simulink library "platooning_custom_blocks"  (R2018b)
settings: Solver=VariableStepAuto  StartTime=0.0  StopTime=10.0  RelTol=1e-3
undefined symbols (not defined in the file): AccPdl_pdlbpt, AccPdl_spdbpt, AccPdl_trqMap, adj_motEffMap, BETModel, BrkPdl_brkTrq, BrkPdl_pdlbpt, Cd_Map, Cd_Map_T2, CT_accPdl_pdlbpt, CT_accPdl_spdbpt, CT_accPdl_trqMap, CT_brkPdl_brkTrq, CT_brkPdl_pdlbpt, CTModel, d_11, d_22, DiscIntNeverNeededParam, init_veh_spd_mps, max_Cd_frac, min_Cd_frac, motSpdVec, motTrqVec, msk_init_pos_m, msk_mot_cont_trq, msk_mot_num, msk_mot_spd_bpt, N_OptResults, sim_t_step, simDrv, SPHETModel, t_step
libraries: simulink x19, $bdroot x16, dspstat3 x2, custom_func x1
(part 3 of 5)

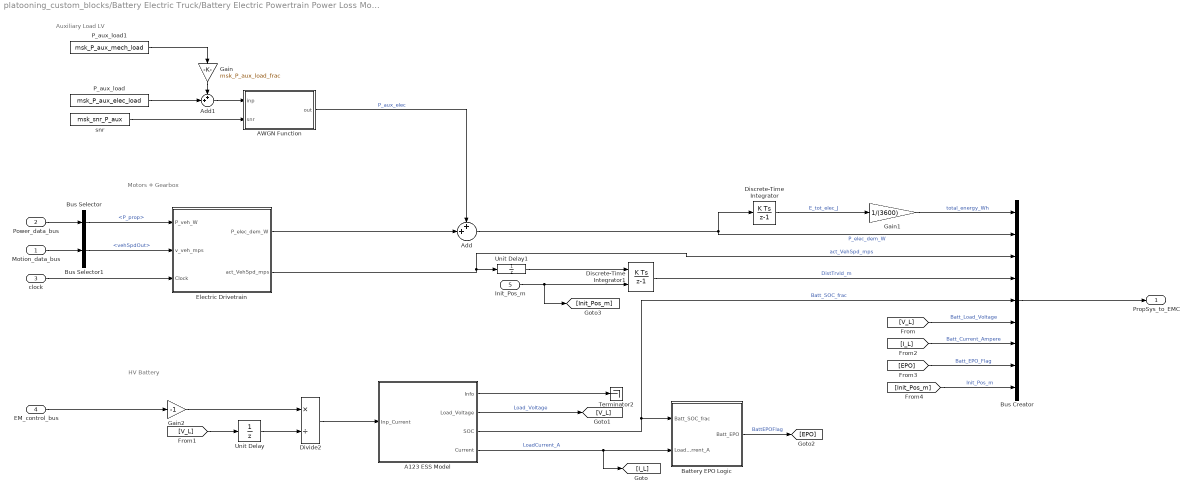
== system platooning_custom_blocks/Battery Electric Truck/Battery Electric Powertrain Power Loss Model ==
  note: Motors + Gearbox
  note: Auxiliary Load LV
  note: HV Battery
  Motion_data_bus : Inport
  Power_data_bus : Inport  Port=2
  clock : Inport  Port=3
  EM_control_bus : Inport  Port=4
  Init_Pos_m : Inport  Port=5
  A123 ESS Model : Subsystem
  AWGN Function : MATLAB Function  TreatAsAtomicUnit=on
  Add : Sum  Inputs=++|
  Add1 : Sum  Inputs=++|
  Battery EPO Logic : Subsystem
  Bus Creator : BusCreator  Inputs=9
  Bus Selector : BusSelector  OutputSignals=P_prop
  Bus Selector1 : BusSelector  OutputSignals=vehSpdOut
  Discrete-Time Integrator : DiscreteIntegrator  SampleTime=msk_t_step  ICPrevOutput=DiscIntNeverNeededParam  ICPrevScaledInput=DiscIntNeverNeededParam
  Discrete-Time Integrator1 : DiscreteIntegrator  InitialConditionSource=external  SampleTime=msk_t_step  ICPrevOutput=DiscIntNeverNeededParam  ICPrevScaledInput=DiscIntNeverNeededParam
  Divide2 : Product  Inputs=*/
  Electric Drivetrain : Subsystem
  Gain : Gain  Gain=msk_P_aux_load_frac
  Gain1 : Gain  Gain=1/(3600)
  Gain2 : Gain  Gain=-1
  P_aux_load : Constant  Value=msk_P_aux_elec_load
  P_aux_load1 : Constant  Value=msk_P_aux_mech_load
  Terminator2 : Terminator
  Unit Delay : UnitDelay  InitialCondition=msk_batt_Ns* msk_batt_Nmod * msk_cell_Vnom  SampleTime=-1
  Unit Delay1 : UnitDelay  SampleTime=-1
  snr : Constant  Value=msk_snr_P_aux
  PropSys_to_EMC : Outport
  wires:
  [Init_Pos_m] -> Bus Creator/9  "Init_Pos_m"
  [EPO] -> Bus Creator/8  "Batt_EPO_Flag"
  [I_L] -> Bus Creator/7  "Batt_Current_Ampere"
  P_aux_load1/1 -> Gain/1
  Gain/1 -> Add1/1
  Add1/1 -> AWGN Function/1(inp)
  Init_Pos_m/1 -> Discrete-Time Integrator1/2, [Init_Pos_m]
  Power_data_bus/1 -> Bus Selector/1
  Motion_data_bus/1 -> Bus Selector1/1
  clock/1 -> Electric Drivetrain/3(Clock)
  Bus Selector1/1 -> Electric Drivetrain/2(v_veh_mps)  "<vehSpdOut>"
  Bus Selector/1 -> Electric Drivetrain/1(P_veh_W)  "<P_prop>"
  P_aux_load/1 -> Add1/2
  snr/1 -> AWGN Function/2(snr)
  AWGN Function/1(out) -> Add/1  "P_aux_elec"
  Add/1 -> Bus Creator/2, Discrete-Time Integrator/1  "P_elec_dem_W"
  Electric Drivetrain/1(P_elec_dem_W) -> Add/2
  Bus Creator/1 -> PropSys_to_EMC/1
  Discrete-Time Integrator/1 -> Gain1/1  "E_tot_elec_J"
  Gain1/1 -> Bus Creator/1  "total_energy_Wh"
  A123 ESS Model/2(Load_Voltage) -> [V_L]  "Load_Voltage"
  Divide2/1 -> A123 ESS Model/1(Inp_Current)
  A123 ESS Model/3(SOC) -> Bus Creator/5, Battery EPO Logic/1(Batt_SOC_frac)  "Batt_SOC_frac"
  A123 ESS Model/1(Info) -> Terminator2/1
  [V_L] -> Unit Delay/1
  Unit Delay/1 -> Divide2/2
  Battery EPO Logic/1(Batt_EPO) -> [EPO]  "BattEPOFlag"
  Gain2/1 -> Divide2/1
  EM_control_bus/1 -> Gain2/1
  A123 ESS Model/4(Current) -> Battery EPO Logic/2(LoadCurrent_A), [I_L]  "LoadCurrent_A"
  Electric Drivetrain/2(act_VehSpd_mps) -> Unit Delay1/1, Bus Creator/3  "act_VehSpd_mps"
  Discrete-Time Integrator1/1 -> Bus Creator/4  "DistTrvld_m"
  Unit Delay1/1 -> Discrete-Time Integrator1/1
  [V_L] -> Bus Creator/6  "Batt_Load_Voltage"

== system platooning_custom_blocks/Battery Electric Truck/Battery Electric Truck Energy Management System ==
  PropSys_to_EMC : Inport
  From_PCL_BUS : Inport  Port=2
  Battery Electric Truck Regen Control Algorithm : MATLAB Function  TreatAsAtomicUnit=on
  Battery Temp degC : Constant  Value=25
  Bus Selector : BusSelector  OutputSignals=P_elec_dem_W,Batt_Load_Voltage,Batt_SOC_frac
  Charge Current Continuous : Lookup_n-D  BreakpointsForDimension1=msk_cell_temp_bpt  BreakpointsForDimension2=msk_soc_bpt  Table=msk_cont_chg_map  InternalRulePriority=Speed  RndMeth=Simplest  InputSameDT=on
  Gain : Gain  Gain=-1
  Multiply : Product
  Terminator : Terminator
  Terminator2 : Terminator
  Unit Delay : UnitDelay  SampleTime=-1
  EMC_to_PropSys : Outport
  wires:
  Bus Selector/2 -> Multiply/1  "<Batt_Load_Voltage>"
  Battery Electric Truck Regen Control Algorithm/1(P_mechbrk_W) -> Terminator2/1
  Charge Current Continuous/1 -> Gain/1
  Battery Electric Truck Regen Control Algorithm/2(P_regenbrk_W) -> EMC_to_PropSys/1  "P_batt_W"
  Bus Selector/1 -> Battery Electric Truck Regen Control Algorithm/1(P_elec_dem)  "<P_elec_dem_W>"
  Bus Selector/3 -> Unit Delay/1  "<Batt_SOC_frac>"
  PropSys_to_EMC/1 -> Bus Selector/1
  From_PCL_BUS/1 -> Terminator/1
  Unit Delay/1 -> Charge Current Continuous/2, Battery Electric Truck Regen Control Algorithm/3(Batt_SOC)
  Multiply/1 -> Battery Electric Truck Regen Control Algorithm/2(P_regen_avail)
  Battery Temp degC/1 -> Charge Current Continuous/1
  Gain/1 -> Multiply/2

== system platooning_custom_blocks/Conventional Truck/Conventional Post-Processing ==
  PropSys_to_EMC : Inport
  Blending Function 1 : Subsystem
  Blending Function 2 : Subsystem
  Bus Creator : BusCreator  Inputs=3
  Bus Creator1 : BusCreator  Inputs=5
  Bus Creator2 : BusCreator  Inputs=3
  Bus Creator3 : BusCreator  Inputs=3
  Bus Selector : BusSelector  OutputSignals=fuelUsed_L,DistTrvld_m,InitPos_m,act_VehSpd_mps,gear_cmd
  Constant1 : Constant  Value=eps
  Distance to Empty Calculator : Subsystem
  Divide1 : Product  Inputs=*/
  Fuel Consumption Calculator : Subsystem
  Fuel LHV energy per volume : Constant  Value=msk_fuel_rho_kgpl * msk_fuel_lhv_kwhpkg
  Product : Product
  Short Term Averaging Function : MATLAB Function  TreatAsAtomicUnit=on
  Short term average distance window - meters : Constant  Value=msk_distwin
  Subtract : Sum  Inputs=+-
  Switch : Switch  Criteria=u2 > Threshold
  kWh2Wh : Gain  Gain=1000
  To_PCL_BUS : Outport
  wires:
  Bus Selector/2 -> Subtract/1, Bus Creator1/2  "<DistTrvld_m>"
  Bus Selector/3 -> Subtract/2  "<InitPos_m>"
  Distance to Empty Calculator/1(estDTE_km) -> Bus Creator1/5  "estDTE_km"
  Constant1/1 -> Switch/3
  Switch/1 -> Divide1/2
  Bus Selector/5 -> Bus Creator1/4  "<gear_cmd>"
  Bus Creator1/1 -> Bus Creator3/3  "State_BUS"
  Subtract/1 -> Fuel Consumption Calculator/2(<DistTrvld_m>), Short Term Averaging Function/3(Dist_Traveled), Switch/2, Switch/1  "DistTrvld_m"
  Divide1/1 -> Blending Function 1/1(runAvgFuelEC_Wh_m), Bus Creator/1  "runAvgElecEC_Wh_m"
  Product/1 -> kWh2Wh/1  "usedFuelEnergy_kWh"
  Short Term Averaging Function/1(STAvg_Wh_m) -> Bus Creator/3, Blending Function 1/3(stAvgFuelEC_Wh_m)  "stAvgElecEC_Wh_m"
  Blending Function 1/1(blndElecEC_Wh_m) -> Bus Creator/2  "blndElecEC_Wh_m"
  Bus Creator/1 -> Bus Creator3/1  "EC_BUS"
  Bus Selector/4 -> Bus Creator1/3  "<act_VehSpd_mps>"
  Fuel LHV energy per volume/1 -> Short Term Averaging Function/2(Fuel_LHV_kWhpL), Product/1
  Short term average distance window - meters/1 -> Short Term Averaging Function/4(Dist_Window)
  PropSys_to_EMC/1 -> Bus Selector/1
  Bus Selector/1 -> Product/2, Fuel Consumption Calculator/1(<fuelUsed_L>), Bus Creator1/1, Distance to Empty Calculator/2(<fuelUsed_L>), Blending Function 2/2(Fuel_Used_L), Blending Function 1/2(Fuel_Used_L), Short Term Averaging Function/1(Fuel_Used_L)  "<fuelUsed_L>"
  kWh2Wh/1 -> Divide1/1
  Short Term Averaging Function/2(STAvg_L_100km) -> Bus Creator2/3, Blending Function 2/3(stAvgFC_L_100km)  "stAvgFC_L_100km"
  Fuel Consumption Calculator/1(FC_Lp100km) -> Bus Creator2/1, Blending Function 2/1(runAvgFC_L_100km)  "runAvgFC_L_100km"
  Blending Function 2/1(blndFC_L_100km) -> Bus Creator2/2, Distance to Empty Calculator/1(blndFC_L_100km)  "blndFC_L_100km"
  Bus Creator2/1 -> Bus Creator3/2  "FC_BUS"
  Bus Creator3/1 -> To_PCL_BUS/1

== system platooning_custom_blocks/Conventional Truck/Conventional Powertrain Energy Management System ==
  PropSys_to_EMC : Inport
  From_PCL_BUS : Inport  Port=2
  Bus Selector : BusSelector  OutputSignals=total_power_W,act_VehSpd_mps
  Optimal Gear Shift Algorithm : $bdroot/Optimal Gear Shift Algorithm  msk_tire_radius_m=CTModel.ld_tire_rad_m  msk_trns_eff_avg=mean(CTModel.gear_eff)  msk_init_gear=1
  Rate Transition : RateTransition  OutPortSampleTime=sim_t_step
  Rate Transition1 : RateTransition  OutPortSampleTime=sim_t_step
  Terminator : Terminator
  EMC_to_PropSys : Outport
  wires:
  Rate Transition1/1 -> Optimal Gear Shift Algorithm/2
  Rate Transition/1 -> Optimal Gear Shift Algorithm/1
  From_PCL_BUS/1 -> Terminator/1
  PropSys_to_EMC/1 -> Bus Selector/1
  Bus Selector/1 -> Rate Transition/1  "<total_power_W>"
  Bus Selector/2 -> Rate Transition1/1  "<act_VehSpd_mps>"
  Optimal Gear Shift Algorithm/1 -> EMC_to_PropSys/1  "opt_gear"

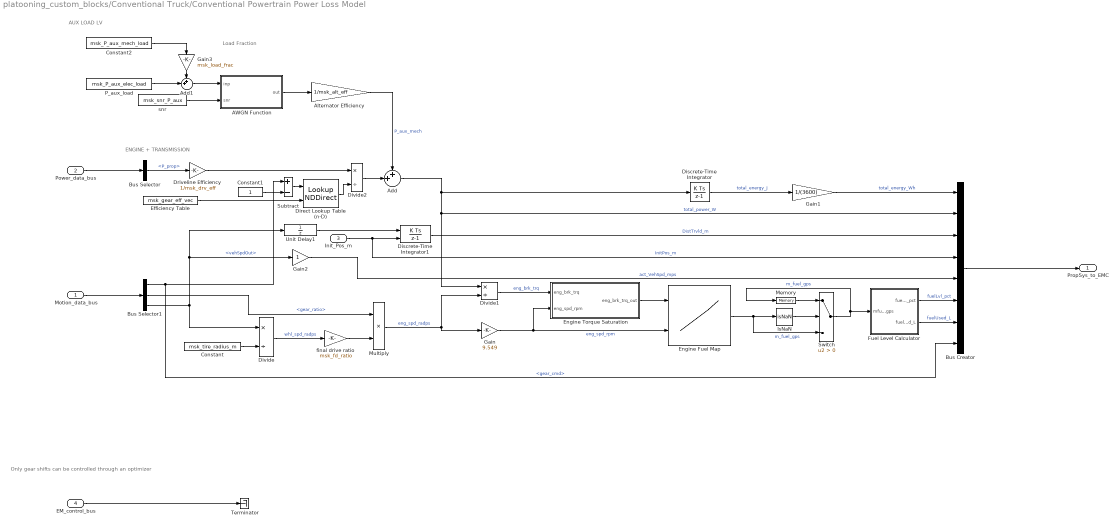
== system platooning_custom_blocks/Conventional Truck/Conventional Powertrain Power Loss Model ==
  note: Only gear shifts can be controlled through an optimizer
  note: ENGINE + TRANSMISSION
  note: AUX LOAD LV
  note: Load Fraction
  Motion_data_bus : Inport
  Power_data_bus : Inport  Port=2
  Init_Pos_m : Inport  Port=3
  EM_control_bus : Inport  Port=4
  AWGN Function : MATLAB Function  TreatAsAtomicUnit=on
  Add : Sum  Inputs=++|
  Add1 : Sum  Inputs=++|
  Alternator Efficiency : Gain  Gain=1/msk_alt_eff
  Bus Creator : BusCreator  Inputs=8
  Bus Selector : BusSelector  OutputSignals=P_prop
  Bus Selector1 : BusSelector  OutputSignals=gear_cmd,gear_ratio,vehSpdOut
  Constant : Constant  Value=msk_tire_radius_m
  Constant1 : Constant
  Constant2 : Constant  Value=msk_P_aux_mech_load
  Direct Lookup Table (n-D) : LookupNDDirect  NumberOfTableDimensions=1  TableIsInput=on
  Discrete-Time Integrator : DiscreteIntegrator  SampleTime=-1  ICPrevOutput=DiscIntNeverNeededParam  ICPrevScaledInput=DiscIntNeverNeededParam
  Discrete-Time Integrator1 : DiscreteIntegrator  InitialConditionSource=external  InitialCondition=msk_init_pos_m  SampleTime=msk_t_step  ICPrevOutput=DiscIntNeverNeededParam  ICPrevScaledInput=DiscIntNeverNeededParam
  Divide : Product  Inputs=*/
  Divide1 : Product  Inputs=*/
  Divide2 : Product  Inputs=*/
  Driveline Efficiency : Gain  Gain=1/msk_drv_eff
  Efficiency Table : Constant  Value=msk_gear_eff_vec
  Engine Fuel Map : Lookup_n-D  BreakpointsForDimension1=msk_eng_trq_bpt  BreakpointsForDimension2=msk_eng_spd_bpt  Table=msk_eng_fuel_map  ExtrapMethod=Clip  UseLastTableValue=on  InternalRulePriority=Speed  RndMeth=Simplest  InputSameDT=on
  Engine Torque Saturation : Subsystem
  Fuel Level Calculator : Subsystem
  Gain : Gain  Gain=9.549
  Gain1 : Gain  Gain=1/(3600)
  Gain2 : Gain
  Gain3 : Gain  Gain=msk_load_frac
  IsNaN : RelationalOperator  Operator=isNaN  OutDataTypeStr=boolean  RndMeth=Simplest
  Memory : Memory
  Multiply : Product
  P_aux_load : Constant  Value=msk_P_aux_elec_load
  Subtract : Sum  Inputs=+-
  Switch : Switch  Criteria=u2 > Threshold
  Terminator : Terminator
  Unit Delay1 : UnitDelay  SampleTime=-1
  final drive ratio : Gain  Gain=msk_fd_ratio
  snr : Constant  Value=msk_snr_P_aux
  PropSys_to_EMC : Outport
  wires:
  P_aux_load/1 -> Add1/2
  Gain3/1 -> Add1/1
  Constant2/1 -> Gain3/1
  Memory/1 -> Switch/1
  IsNaN/1 -> Switch/2
  Engine Fuel Map/1 -> IsNaN/1, Switch/3  "m_fuel_gps"
  Power_data_bus/1 -> Bus Selector/1
  Motion_data_bus/1 -> Bus Selector1/1
  Init_Pos_m/1 -> Discrete-Time Integrator1/2, Bus Creator/4  "InitPos_m"
  EM_control_bus/1 -> Terminator/1
  Bus Selector1/3 -> Gain2/1, Unit Delay1/1, Divide/1  "<vehSpdOut>"
  Bus Selector/1 -> Driveline Efficiency/1  "<P_prop>"
  Add1/1 -> AWGN Function/1(inp)
  snr/1 -> AWGN Function/2(snr)
  AWGN Function/1(out) -> Alternator Efficiency/1
  Alternator Efficiency/1 -> Add/1  "P_aux_mech"
  Switch/1 -> Fuel Level Calculator/1(mfuel_gps), Memory/1  "m_fuel_gps"
  Constant/1 -> Divide/2
  Divide/1 -> final drive ratio/1  "whl_spd_radps"
  final drive ratio/1 -> Multiply/2
  Multiply/1 -> Divide1/2, Gain/1  "eng_spd_radps"
  Gain/1 -> Engine Torque Saturation/2(eng_spd_rpm), Engine Fuel Map/2  "eng_spd_rpm"
  Add/1 -> Bus Creator/2, Divide1/1, Discrete-Time Integrator/1  "total_power_W"
  Divide2/1 -> Add/2
  Bus Selector1/2 -> Multiply/1  "<gear_ratio>"
  Bus Creator/1 -> PropSys_to_EMC/1
  Discrete-Time Integrator/1 -> Gain1/1  "total_energy_J"
  Fuel Level Calculator/1(fuelLvl_pct) -> Bus Creator/6  "fuelLvl_pct"
  Fuel Level Calculator/2(fuelUsed_L) -> Bus Creator/7  "fuelUsed_L"
  Gain1/1 -> Bus Creator/1  "total_energy_Wh"
  Divide1/1 -> Engine Torque Saturation/1(eng_brk_trq)  "eng_brk_trq"
  Engine Torque Saturation/1(eng_brk_trq_out) -> Engine Fuel Map/1
  Unit Delay1/1 -> Discrete-Time Integrator1/1
  Discrete-Time Integrator1/1 -> Bus Creator/3  "DistTrvld_m"
  Gain2/1 -> Bus Creator/5  "act_VehSpd_mps"
  Driveline Efficiency/1 -> Divide2/1
  Efficiency Table/1 -> Direct Lookup Table (n-D)/2
  Direct Lookup Table (n-D)/1 -> Divide2/2
  Subtract/1 -> Direct Lookup Table (n-D)/1
  Constant1/1 -> Subtract/2
  Bus Selector1/1 -> Bus Creator/8, Subtract/1  "<gear_cmd>"

== system platooning_custom_blocks/Series Parallel Hybrid Electric Truck/Series Parallel Hybrid Electric Post-Processing ==
  PropSys_to_EMC : Inport
  Add : Sum
  Battery Energy Max : Constant  Value=msk_batt_Ns * msk_batt_Np * msk_batt_Nmod * msk_cell_Vnom * msk_cell_Q_Ah
  Blending Function 1 : Subsystem
  Blending Function 2 : Subsystem
  Bus Creator1 : BusCreator  Inputs=11
  Bus Creator2 : BusCreator  Inputs=3
  Bus Creator3 : BusCreator  Inputs=3
  Bus Creator5 : BusCreator  Inputs=3
  Bus Selector : BusSelector  OutputSignals=Batt_Voltage_V,Batt_EPO_Flag,Batt_Current_A,P_gen_mech_W,GearCmd,eng_spd_rpm,Batt_SOC_frac,DistTrvld_m,Init_Pos_m,act_VehSpd_mps,fuelUsed_L
  Constant : Constant  Value=msk_batt_soc_init
  Constant2 : Constant  Value=eps
  Distance to Empty Calculator : Subsystem
  Divide1 : Product  Inputs=*/
  Fuel Consumption Calculator : Subsystem
  Fuel LHV energy per volume : Constant  Value=msk_fuel_rho_kgpl * msk_fuel_lhv_kwhpkg
  Product : Product
  Product1 : Product
  Short Term Averaging Function1 : MATLAB Function  TreatAsAtomicUnit=on
  Short term average distance window - meters1 : Constant  Value=msk_distwin
  Subtract : Sum  Inputs=+-
  Subtract1 : Sum  Inputs=+-
  Switch : Switch  Criteria=u2 > Threshold
  kWh2Wh : Gain  Gain=1000
  To_PCL_BUS : Outport
  wires:
  Bus Selector/8 -> Subtract1/1, Bus Creator1/8  "<DistTrvld_m>"
  Bus Selector/9 -> Subtract1/2  "<Init_Pos_m>"
  Bus Selector/6 -> Bus Creator1/6  "<eng_spd_rpm>"
  Bus Selector/5 -> Bus Creator1/5  "<GearCmd>"
  Bus Selector/4 -> Bus Creator1/4  "<P_gen_mech_W>"
  Bus Selector/3 -> Bus Creator1/3  "<Batt_Current_A>"
  Bus Selector/2 -> Bus Creator1/2  "<Batt_EPO_Flag>"
  Bus Selector/1 -> Bus Creator1/1  "<Batt_Voltage_V>"
  Distance to Empty Calculator/1(estDTE_km) -> Bus Creator1/11  "estDTE_km"
  Constant2/1 -> Switch/3
  Switch/1 -> Divide1/2
  PropSys_to_EMC/1 -> Bus Selector/1
  Bus Selector/7 -> Bus Creator1/7, Distance to Empty Calculator/3(battSOC_frac), Short Term Averaging Function1/1(Batt_SOC_frac), Subtract/2  "<Batt_SOC_frac>"
  Constant/1 -> Subtract/1
  Subtract/1 -> Product/2
  Product/1 -> Add/1  "total_elec_Energy_Wh"
  Battery Energy Max/1 -> Short Term Averaging Function1/2(Batt_Max_Energy), Product/1
  Bus Creator1/1 -> Bus Creator2/1  "State_BUS"
  Bus Creator2/1 -> To_PCL_BUS/1
  Bus Creator5/1 -> Bus Creator2/3  "FC_BUS"
  Product1/1 -> kWh2Wh/1  "usedFuelEnergy_kWh"
  Blending Function 2/1(blndFC_L_100km) -> Bus Creator5/2  "blndFC_L_100km"
  Divide1/1 -> Blending Function 1/1(runAvgFuelEC_Wh_m), Bus Creator3/1  "runAvgElecEC_Wh_m"
  Bus Selector/10 -> Bus Creator1/9  "<act_VehSpd_mps>"
  Short Term Averaging Function1/1(STAvg_Wh_m) -> Blending Function 1/3(stAvgFuelEC_Wh_m), Bus Creator3/3  "stAvgElecEC_Wh_m"
  Bus Creator3/1 -> Bus Creator2/2  "EC_BUS"
  Short term average distance window - meters1/1 -> Short Term Averaging Function1/6(Dist_Window)
  Blending Function 1/1(blndElecEC_Wh_m) -> Bus Creator3/2, Distance to Empty Calculator/1(blndEC_Wh_m)  "blndElecEC_Wh_m"
  kWh2Wh/1 -> Add/2
  Subtract1/1 -> Switch/2, Switch/1, Fuel Consumption Calculator/2(<DistTrvld_m>), Short Term Averaging Function1/5(Dist_Traveled)  "DistTrvld_m"
  Short Term Averaging Function1/2(STAvg_L_100km) -> Bus Creator5/3, Blending Function 2/3(stAvgFC_L_100km)  "stAvgFC_L_100km"
  Fuel LHV energy per volume/1 -> Short Term Averaging Function1/4(Fuel_LHV_kWhpL), Product1/1
  Fuel Consumption Calculator/1(FC_Lp100km) -> Bus Creator5/1, Blending Function 2/1(runAvgFC_L_100km)  "runAvgFC_L_100km"
  Bus Selector/11 -> Product1/2, Distance to Empty Calculator/2(<fuelUsed_L>), Blending Function 1/2(Fuel_Used_L), Blending Function 2/2(Fuel_Used_L), Short Term Averaging Function1/3(Fuel_Used_L), Fuel Consumption Calculator/1(<fuelUsed_L>), Bus Creator1/10  "<fuelUsed_L>"
  Add/1 -> Divide1/1

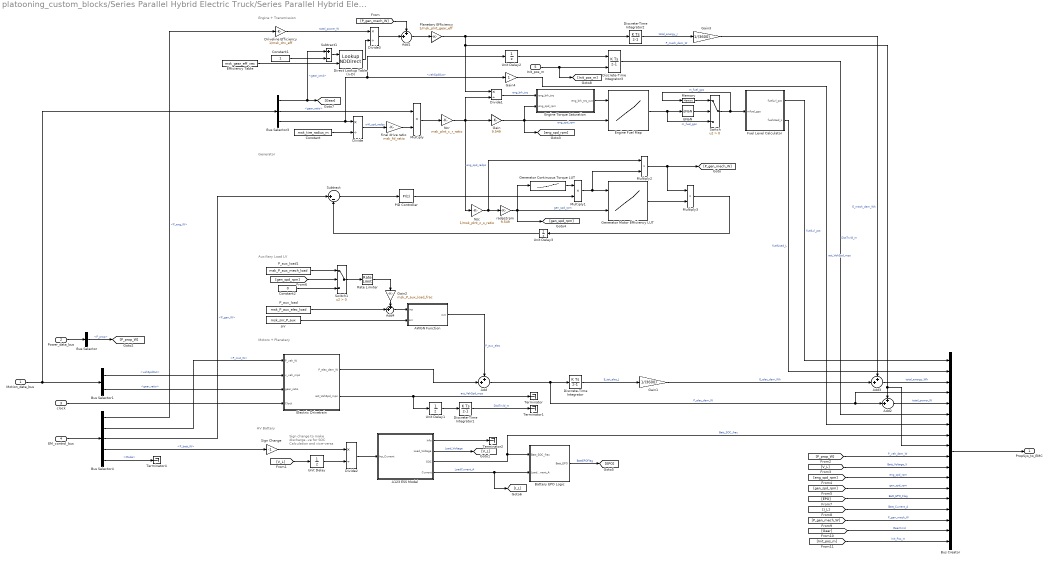
== system platooning_custom_blocks/Series Parallel Hybrid Electric Truck/Series Parallel Hybrid Electric Powertrain Power Loss Model ==
  note: Generator
  note: Motors + Planetary
  note: Auxiliary Load LV
  note: HV Battery
  note: Engine + Transmission
  note: Sign change to make discharge -ve
      | for SOC Calculation and vice-versa
  Motion_data_bus : Inport
  Power_data_bus : Inport  Port=2
  clock : Inport  Port=3
  EM_control_bus : Inport  Port=4
  Init_pos_m : Inport  Port=5
  A123 ESS Model : Subsystem
  AWGN Function : MATLAB Function  TreatAsAtomicUnit=on
  Add{,1..4} (5 alike) : Sum  Inputs=++|
  Battery EPO Logic : Subsystem
  Bus Creator : BusCreator  Inputs=18
  Bus Selector : BusSelector  OutputSignals=P_prop
  Bus Selector1 : BusSelector  OutputSignals=vehSpdOut,gear_ratio
  Bus Selector3 : BusSelector  OutputSignals=gear_cmd,gear_ratio,vehSpdOut
  Bus Selector4 : BusSelector  OutputSignals=P_eng_W,P_mot_W,P_gen_W,P_batt_W,Mode
  Constant : Constant  Value=msk_tire_radius_m
  Constant1 : Constant
  Constant2 : Constant  Value=0
  Direct Lookup Table (n-D) : LookupNDDirect  NumberOfTableDimensions=1  TableIsInput=on
  Discrete-Time Integrator : DiscreteIntegrator  SampleTime=msk_t_step  ICPrevOutput=DiscIntNeverNeededParam  ICPrevScaledInput=DiscIntNeverNeededParam
  Discrete-Time Integrator1 : DiscreteIntegrator  SampleTime=msk_t_step  ICPrevOutput=DiscIntNeverNeededParam  ICPrevScaledInput=DiscIntNeverNeededParam
  Discrete-Time Integrator2 : DiscreteIntegrator  SampleTime=-1  ICPrevOutput=DiscIntNeverNeededParam  ICPrevScaledInput=DiscIntNeverNeededParam
  Discrete-Time Integrator3 : DiscreteIntegrator  InitialConditionSource=external  SampleTime=msk_t_step  ICPrevOutput=DiscIntNeverNeededParam  ICPrevScaledInput=DiscIntNeverNeededParam
  Divide{,1..3} (4 alike) : Product  Inputs=*/
  Driveline Efficiency : Gain  Gain=1/msk_drv_eff
  Efficiency Table : Constant  Value=msk_gear_eff_vec
  Electric Drivetrain : Subsystem
  Engine Fuel Map : Lookup_n-D  BreakpointsForDimension1=msk_eng_trq_bpt  BreakpointsForDimension2=msk_eng_spd_bpt  Table=msk_eng_fuel_map  ExtrapMethod=Clip  UseLastTableValue=on  InternalRulePriority=Speed  RndMeth=Simplest  InputSameDT=on
  Engine Torque Saturation : Subsystem
  Fuel Level Calculator : Subsystem
  Gain : Gain  Gain=9.549
  Gain1 : Gain  Gain=1/(3600)
  Gain2 : Gain  Gain=msk_P_aux_load_frac
  Gain3 : Gain  Gain=1/(3600)
  Gain4 : Gain
  Generator Continuous Torque LUT : Lookup_n-D  NumberOfTableDimensions=1  BreakpointsForDimension1=msk_gen_mtr_spdbpt  Table=msk_gen_mtr_cont_trq  InternalRulePriority=Speed  RndMeth=Simplest  InputSameDT=on
  Generator Motor Efficiency LUT : Lookup_n-D  BreakpointsForDimension1=msk_gen_mtr_trqbpt  BreakpointsForDimension2=msk_gen_mtr_spdbpt  Table=msk_gen_mtr_eff_map  ExtrapMethod=Clip  UseLastTableValue=on  InternalRulePriority=Speed  RndMeth=Simplest  InputSameDT=on
  IsNaN : RelationalOperator  Operator=isNaN  OutDataTypeStr=boolean  RndMeth=Simplest
  Memory : Memory
  Multiply{,1..3} (4 alike) : Product
  Ncr : Gain  Gain=msk_plnt_c_r_ratio
  Nsc : Gain  Gain=1/msk_plnt_c_s_ratio
  PID Controller : simulink/Continuous/PID Controller  Controller=PI  Form=Parallel  TimeDomain=Discrete-time  SampleTime=-1  IntegratorMethod=Forward Euler  FilterMethod=Forward Euler  ControllerParametersSource=internal  P=msk_gen_ctl_Kp  I=msk_gen_ctl_Ki  D=0  UseFilter=on  N=100  TunerSelectOption=Transfer Function Based (PID Tuner App)  InitialConditionSource=internal  InitialConditionForIntegrator=0  InitialConditionForFilter=0  DifferentiatorICPrevScaledInput=0  ExternalReset=none  TrackingMode=off  Kt=1  LimitOutput=on  UpperSaturationLimit=1  LowerSaturationLimit=0  LinearizeAsGain=on  AntiWindupMode=clamping  Kb=1  POutMin=[]  POutMax=[]  IOutMin=[]  IOutMax=[]  DOutMin=[]  DOutMax=[]  NOutMin=[]  NOutMax=[]  SumOutMin=[]  SumOutMax=[]  SaturationOutMin=[]  SaturationOutMax=[]  PParamMin=[]  PParamMax=[]  IParamMin=[]  IParamMax=[]  DParamMin=[]  DParamMax=[]  NParamMin=[]  NParamMax=[]  KbParamMin=[]  KbParamMax=[]  KtParamMin=[]  KtParamMax=[]  KbOutMin=[]  KbOutMax=[]  KtOutMin=[]  KtOutMax=[]  IntegratorOutMin=[]  IntegratorOutMax=[]  FilterOutMin=[]  FilterOutMax=[]  SumI1OutMin=[]  SumI1OutMax=[]  SumI2OutMin=[]  SumI2OutMax=[]  SumI3OutMin=[]  SumI3OutMax=[]  SumI4OutMin=[]  SumI4OutMax=[]  SumDOutMin=[]  SumDOutMax=[]  DifferentiatorOutMin=[]  DifferentiatorOutMax=[]  FilterDiffOutCoefMin=[]  FilterDiffOutCoefMax=[]  ReciprocalOutMin=[]  ReciprocalOutMax=[]  SumDenOutMin=[]  SumDenOutMax=[]  SumNumOutMin=[]  SumNumOutMax=[]  DivideOutMin=[]  DivideOutMax=[]  IntegratorContinuousStateAttributes=''  IntegratorStateMustResolveToSignalObject=off  IntegratorRTWStateStorageClass=Auto  FilterContinuousStateAttributes=''  FilterStateMustResolveToSignalObject=off  FilterRTWStateStorageClass=Auto  ParallelPVariant=InternalParameters  IdealPVariant=Disabled  IVariant=InternalParameters  DVariant=Disabled  IntegratorVariant=Discrete  SatVariant=Enabled  AWVariant=DiscClampingParallel  PCopyVariant=Disabled  TRVariant=Disabled  FdbkBlocksVariant=Forward  IdealPFdbkVariant=Disabled  SatFdbkVariant=Disabled  DerivativeFilterVariant=Disabled  NVariant=Disabled  NCopyVariant=Disabled_SignalSpec  FilterICVariant=Disabled  IntegratorICVariant=InternalICs  ExternalResetVariant=Disabled  TRSumVariant=Passthrough  SumFdbkVariant=Disabled  SumVariant=Sum_PI
  P_aux_load : Constant  Value=msk_P_aux_elec_load
  P_aux_load1 : Constant  Value=msk_P_aux_mech_load
  Planetary Efficiency : Gain  Gain=1/msk_plnt_gear_eff
  Rate Limiter : RateLimiter  RisingSlewLimit=100  FallingSlewLimit=-100  SampleTimeMode=inherited
  Sign Change : Gain  Gain=-1
  Subtract : Sum  Inputs=|+-
  Subtract1 : Sum  Inputs=+-
  Switch : Switch  Criteria=u2 > Threshold
  Switch1 : Switch  Criteria=u2 > Threshold
  Terminator{,1..2,4} (4 alike) : Terminator
  Unit Delay : UnitDelay  InitialCondition=msk_batt_Ns* msk_batt_Nmod * msk_cell_Vnom  SampleTime=-1
  Unit Delay1 : UnitDelay  SampleTime=-1
  Unit Delay2 : UnitDelay  SampleTime=-1
  Unit Delay3 : UnitDelay  SampleTime=-1
  final drive ratio : Gain  Gain=msk_fd_ratio
  radps2rpm : Gain  Gain=9.549
  snr : Constant  Value=msk_snr_P_aux
  PropSys_to_EMC : Outport
  wires:
  [Init_pos_m] -> Bus Creator/18  "Init_Pos_m"
  Planetary Efficiency/1 -> Discrete-Time Integrator2/1, Add2/1, Bus Creator/9, Divide1/1  "P_mech_dem_W"
  [P_gen_mech_W] -> Bus Creator/16  "P_gen_mech_W"
  [I_L] -> Bus Creator/15  "Batt_Current_A"
  [EPO] -> Bus Creator/14  "Batt_EPO_Flag"
  [Gear] -> Bus Creator/17  "GearCmd"
  Constant2/1 -> Switch1/3
  [gen_spd_rpm] -> Switch1/2
  Rate Limiter/1 -> Gain2/1
  Switch1/1 -> Rate Limiter/1
  P_aux_load1/1 -> Switch1/1
  Gain2/1 -> Add4/1
  Add4/1 -> AWGN Function/1(inp)
  Init_pos_m/1 -> Discrete-Time Integrator3/2, [Init_pos_m]
  [eng_spd_rpm] -> Bus Creator/12  "eng_spd_rpm"
  [gen_spd_rpm] -> Bus Creator/13  "gen_spd_rpm"
  Ncr/1 -> Nsc/1, Gain/1, Divide1/2  "eng_spd_radps"
  [V_L] -> Bus Creator/11  "Batt_Voltage_V"
  Bus Selector4/5 -> Terminator4/1  "<Mode>"
  Bus Selector4/3 -> Subtract/1  "<P_gen_W>"
  Bus Selector4/1 -> Driveline Efficiency/1  "<P_eng_W>"
  [P_prop_W] -> Bus Creator/10  "P_veh_dem_W"
  IsNaN/1 -> Switch/2
  Engine Fuel Map/1 -> IsNaN/1, Switch/3  "m_fuel_gps"
  Memory/1 -> Switch/1
  Switch/1 -> Memory/1, Fuel Level Calculator/1(mfuel_gps)  "m_fuel_gps"
  Bus Selector3/1 -> [Gear], Subtract1/1  "<gear_cmd>"
  Power_data_bus/1 -> Bus Selector/1
  clock/1 -> Electric Drivetrain/4(Clock)
  Bus Selector1/1 -> Electric Drivetrain/2(v_veh_mps)  "<vehSpdOut>"
  P_aux_load/1 -> Add4/2
  snr/1 -> AWGN Function/2(snr)
  AWGN Function/1(out) -> Add/1  "P_aux_elec"
  Add/1 -> Discrete-Time Integrator/1, Add2/2, Bus Creator/4  "P_elec_dem_W"
  Electric Drivetrain/1(P_elec_dem_W) -> Add/2
  Bus Creator/1 -> PropSys_to_EMC/1
  Discrete-Time Integrator/1 -> Gain1/1  "E_tot_elec_J"
  Gain1/1 -> Add3/2  "E_elec_dem_Wh"
  A123 ESS Model/2(Load_Voltage) -> [V_L]  "Load_Voltage"
  Divide2/1 -> A123 ESS Model/1(Inp_Current)
  A123 ESS Model/3(SOC) -> Bus Creator/8, Battery EPO Logic/1(Batt_SOC_frac)  "Batt_SOC_frac"
  A123 ESS Model/1(Info) -> Terminator2/1
  [V_L] -> Unit Delay/1
  Unit Delay/1 -> Divide2/2
  Battery EPO Logic/1(Batt_EPO) -> [EPO]  "BattEPOFlag"
  Sign Change/1 -> Divide2/1
  Bus Selector4/4 -> Sign Change/1  "<P_batt_W>"
  A123 ESS Model/4(Current) -> Battery EPO Logic/2(LoadCurrent_A), [I_L]  "LoadCurrent_A"
  Electric Drivetrain/2(act_VehSpd_mps) -> Terminator/1, Unit Delay1/1  "act_VehSpd_mps"
  Discrete-Time Integrator1/1 -> Terminator1/1  "DistTrvld_m"
  Unit Delay1/1 -> Discrete-Time Integrator1/1
  Gain/1 -> Engine Torque Saturation/2(eng_spd_rpm), Engine Fuel Map/2, [eng_spd_rpm]  "eng_spd_rpm"
  Constant/1 -> Divide/2
  Gain3/1 -> Add3/1  "E_mech_dem_Wh"
  Motion_data_bus/1 -> Bus Selector3/1, Bus Selector1/1
  Fuel Level Calculator/1(fuelLvl_pct) -> Bus Creator/1  "fuelLvl_pct"
  Engine Torque Saturation/1(eng_brk_trq_out) -> Engine Fuel Map/1
  Discrete-Time Integrator2/1 -> Gain3/1  "total_energy_J"
  Multiply/1 -> Ncr/1
  Fuel Level Calculator/2(fuelUsed_L) -> Bus Creator/2  "fuelUsed_L"
  Divide1/1 -> Engine Torque Saturation/1(eng_brk_trq)  "eng_brk_trq"
  Discrete-Time Integrator3/1 -> Bus Creator/6  "DistTrvld_m"
  Gain4/1 -> Bus Creator/7  "act_VehSpd_mps"
  Divide/1 -> final drive ratio/1  "whl_spd_radps"
  Bus Selector3/3 -> Gain4/1, Unit Delay2/1, Divide/1  "<vehSpdOut>"
  Unit Delay2/1 -> Discrete-Time Integrator3/1
  final drive ratio/1 -> Multiply/2
  EM_control_bus/1 -> Bus Selector4/1
  Bus Selector/1 -> [P_prop_W]  "<P_prop>"
  Bus Selector4/2 -> Electric Drivetrain/1(P_veh_W)  "<P_mot_W>"
  Nsc/1 -> Multiply2/1, radps2rpm/1
  radps2rpm/1 -> Generator Continuous Torque LUT/1, Generator Motor Efficiency LUT/2, [gen_spd_rpm]  "gen_spd_rpm"
  Subtract/1 -> PID Controller/1
  PID Controller/1 -> Multiply1/2
  Multiply1/1 -> Multiply2/2, Generator Motor Efficiency LUT/1
  Generator Continuous Torque LUT/1 -> Multiply1/1
  Generator Motor Efficiency LUT/1 -> Multiply3/2
  Multiply2/1 -> [P_gen_mech_W], Multiply3/1
  Multiply3/1 -> Unit Delay3/1
  Unit Delay3/1 -> Subtract/2
  [P_gen_mech_W] -> Add1/1
  Driveline Efficiency/1 -> Divide3/1  "total_power_W"
  Bus Selector1/2 -> Electric Drivetrain/3(gear_ratio)  "<gear_ratio>"
  Add1/1 -> Planetary Efficiency/1
  Add2/1 -> Bus Creator/5  "total_power_W"
  Add3/1 -> Bus Creator/3  "total_energy_Wh"
  Subtract1/1 -> Direct Lookup Table (n-D)/1
  Constant1/1 -> Subtract1/2
  Efficiency Table/1 -> Direct Lookup Table (n-D)/2
  Direct Lookup Table (n-D)/1 -> Divide3/2
  Bus Selector3/2 -> Multiply/1  "<gear_ratio>"
  Divide3/1 -> Add1/2

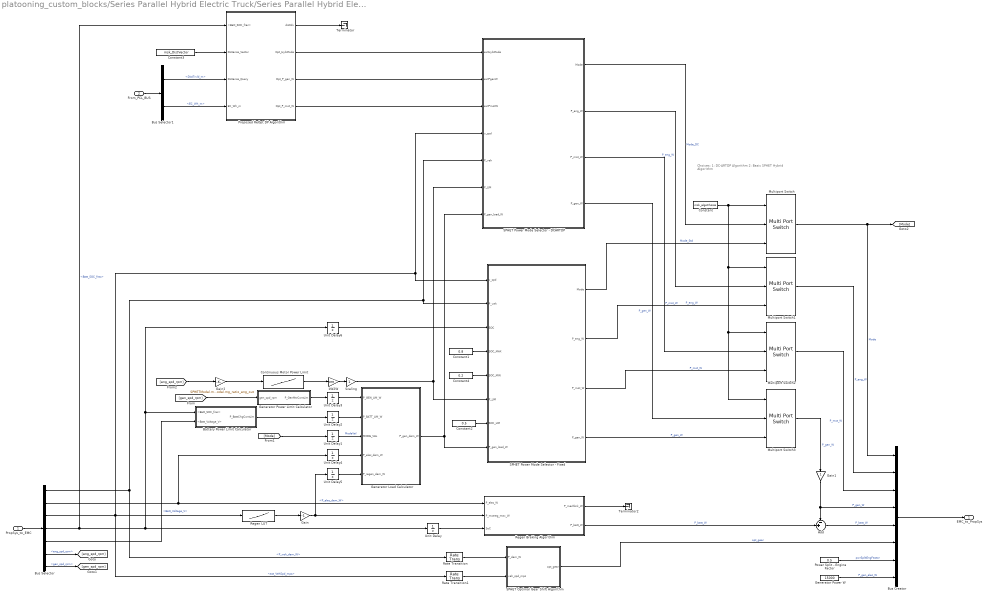
== system platooning_custom_blocks/Series Parallel Hybrid Electric Truck/Series Parallel Hybrid Electric Truck Energy Management System ==
  note: Choices:
      | 1: DC-ARTDP Algorithm
      | 2: Basic SPHET Hybrid Algorithm
  PropSys_to_EMC : Inport
  From_PCL_BUS : Inport  Port=2
  Add : Sum  Inputs=-+|
  Battery Power Limit Calculator : Subsystem
  Bus Creator : BusCreator  Inputs=8
  Bus Selector : BusSelector  OutputSignals=P_veh_dem_W,P_elec_dem_W,act_VehSpd_mps,Batt_SOC_frac,Batt_Voltage_V,eng_spd_rpm,gen_spd_rpm
  Bus Selector1 : BusSelector  OutputSignals=DistTrvld_m,EC_Wh_m
  Constant : Constant  Value=msk_algoChoice
  Constant1 : Constant  Value=0.8
  Constant2 : Constant  Value=0.5
  Constant3 : Constant  Value=msk_DistVector
  Constant4 : Constant  Value=0.2
  Continuous Motor Power Limit : Lookup_n-D  NumberOfTableDimensions=1  BreakpointsForDimension1=SPHETModel.cont_mtr_trq_spdbpt  Table=SPHETModel.cont_mtr_pwr_map  InternalRulePriority=Speed  RndMeth=Simplest  InputSameDT=on
  Gain : Gain  Gain=-1
  Gain1 : Gain
  Gain2 : Gain  Gain=SPHETModel.mg_ratio_mot_out/SPHETModel.mg_ratio_eng_out
  Generator Load Calculator : MATLAB Function  TreatAsAtomicUnit=on
  Generator Power Limit Calculator : Subsystem
  Generator Power W : Constant  Value=15000
  Multiport Switch{,1..3} (4 alike) : MultiPortSwitch  Inputs=2
  Power Split - Engine Factor : Constant  Value=0.5
  Proposed ReOpt DP Algorithm : Subsystem
  Rate Transition : RateTransition  OutPortSampleTime=sim_t_step
  Rate Transition1 : RateTransition  OutPortSampleTime=sim_t_step
  Regen Braking Algorithm : Stateflow chart  TreatAsAtomicUnit=on
  Regen LUT : Lookup_n-D  NumberOfTableDimensions=1  BreakpointsForDimension1=msk_regen_spd_bpt  Table=msk_regen_pwr_vec*-1  ExtrapMethod=Clip  UseLastTableValue=on  InternalRulePriority=Speed  RndMeth=Simplest  InputSameDT=on
  SPHET Optimal Gear Shift Algorithm : Subsystem  mask{msk_tire_radius_m=SPHETModel.ld_tire_rad_m, msk_trns_eff_avg=mean(SPHETModel.gear_eff) * SPHETModel.plnt_gear_eff, msk_init_gear=1}
      mask prompts: msk_tire_radius_m "Vehicle tire radius :"; msk_trns_eff_avg "Average transmission efficiency :"; msk_init_gear "Initial gear selection :"
      mask DialogControl DescGroupVar Prompt: Optimal Gear Shift Algorithm
      mask DialogControl DescTextVar Prompt: The block computes optimal gear based on the power demand and vehicle speed by minimizing fuel consumption.
  SPHET Power Mode Selector - DCARTDP : Stateflow chart  TreatAsAtomicUnit=on
  SPHET Power Mode Selector - Fixed : Stateflow chart  TreatAsAtomicUnit=on
  Scaling : Gain
  Terminator : Terminator
  Terminator2 : Terminator
  Unit Delay{,1..6} (7 alike) : UnitDelay  SampleTime=-1
  kW2W : Gain  Gain=1000
  EMC_to_PropSys : Outport
  wires:
  Constant4/1 -> SPHET Power Mode Selector - Fixed/5(SOC_MIN)
  Scaling/1 -> SPHET Power Mode Selector - Fixed/6(P_LIM), SPHET Power Mode Selector - DCARTDP/6(P_LIM)
  Constant3/1 -> Proposed ReOpt DP Algorithm/2(Distance_Vector)
  Proposed ReOpt DP Algorithm/1(distIdx) -> Terminator/1
  Proposed ReOpt DP Algorithm/3(Opt_P_gen_W) -> SPHET Power Mode Selector - DCARTDP/2(extPgenW)
  Proposed ReOpt DP Algorithm/2(Opt_HybMode) -> SPHET Power Mode Selector - DCARTDP/1(extHybMode)
  Proposed ReOpt DP Algorithm/4(Opt_P_mot_W) -> SPHET Power Mode Selector - DCARTDP/3(extPmotW)
  Bus Selector1/1 -> Proposed ReOpt DP Algorithm/3(Distance_Query)  "<DistTrvld_m>"
  Bus Selector1/2 -> Proposed ReOpt DP Algorithm/4(EC_Wh_m)  "<EC_Wh_m>"
  Constant/1 -> Multiport Switch/1, Multiport Switch1/1, Multiport Switch2/1, Multiport Switch3/1
  SPHET Power Mode Selector - DCARTDP/1(Mode) -> Multiport Switch/2  "Mode_DC"
  SPHET Power Mode Selector - DCARTDP/2(P_eng_W) -> Multiport Switch1/2  "P_eng_W"
  SPHET Power Mode Selector - DCARTDP/3(P_mot_W) -> Multiport Switch2/2  "P_mot_W"
  SPHET Power Mode Selector - DCARTDP/4(P_gen_W) -> Multiport Switch3/2  "P_gen_W"
  SPHET Power Mode Selector - Fixed/1(Mode) -> Multiport Switch/3  "Mode_Std"
  SPHET Power Mode Selector - Fixed/2(P_eng_W) -> Multiport Switch1/3  "P_eng_W"
  SPHET Power Mode Selector - Fixed/3(P_mot_W) -> Multiport Switch2/3  "P_mot_W"
  SPHET Power Mode Selector - Fixed/4(P_gen_W) -> Multiport Switch3/3  "P_gen_W"
  [eng_spd_rpm] -> Gain2/1
  Gain2/1 -> Continuous Motor Power Limit/1
  Continuous Motor Power Limit/1 -> kW2W/1
  Unit Delay6/1 -> SPHET Power Mode Selector - Fixed/3(SOC)
  Unit Delay5/1 -> Generator Load Calculator/5(P_regen_dem_W)
  Unit Delay4/1 -> Generator Load Calculator/4(P_elec_dem_W)
  Unit Delay3/1 -> Generator Load Calculator/1(P_GEN_LIM_W)
  Unit Delay2/1 -> Generator Load Calculator/2(P_BATT_LIM_W)
  Gain1/1 -> Bus Creator/4, Add/1  "P_gen_W"
  Gain/1 -> Unit Delay5/1, Regen Braking Algorithm/2(P_motreg_max_W)
  Generator Power Limit Calculator/1(P_GenMtrContLim) -> Unit Delay3/1
  [gen_spd_rpm] -> Generator Power Limit Calculator/1(gen_spd_rpm)
  Battery Power Limit Calculator/1(P_BattChgContLim) -> Unit Delay2/1
  Bus Selector/5 -> Battery Power Limit Calculator/2(<Batt_Voltage_V>)  "<Batt_Voltage_V>"
  Unit Delay1/1 -> Generator Load Calculator/3(MODE_VAL)  "ModeVal"
  [Mode] -> Unit Delay1/1
  Bus Selector/7 -> [gen_spd_rpm]  "<gen_spd_rpm>"
  Bus Selector/6 -> [eng_spd_rpm]  "<eng_spd_rpm>"
  Generator Load Calculator/1(P_gen_dem_W) -> SPHET Power Mode Selector - Fixed/8(P_gen_load_W), SPHET Power Mode Selector - DCARTDP/7(P_gen_load_W)
  Multiport Switch2/1 -> Bus Creator/3  "P_mot_W"
  Multiport Switch1/1 -> Bus Creator/2  "P_eng_W"
  Multiport Switch3/1 -> Gain1/1  "P_gen_W"
  Regen Braking Algorithm/2(P_batt_W) -> Add/2  "P_batt_W"
  Multiport Switch/1 -> [Mode], Bus Creator/1  "Mode"
  Constant2/1 -> SPHET Power Mode Selector - Fixed/7(SOC_LIM)
  Constant1/1 -> SPHET Power Mode Selector - Fixed/4(SOC_MAX)
  kW2W/1 -> Scaling/1
  SPHET Optimal Gear Shift Algorithm/1(opt_gear) -> Bus Creator/6  "opt_gear"
  Rate Transition1/1 -> SPHET Optimal Gear Shift Algorithm/2(veh_spd_mps)
  Rate Transition/1 -> SPHET Optimal Gear Shift Algorithm/1(P_dem_W)
  Bus Selector/3 -> Rate Transition1/1, SPHET Power Mode Selector - Fixed/1(v_spd), SPHET Power Mode Selector - DCARTDP/4(v_spd), Regen LUT/1  "<act_VehSpd_mps>"
  Unit Delay/1 -> Regen Braking Algorithm/3(SoC)
  Regen Braking Algorithm/1(P_mechbrk_W) -> Terminator2/1
  Regen LUT/1 -> Gain/1
  Add/1 -> Bus Creator/5  "P_batt_W"
  Bus Selector/2 -> Unit Delay4/1, Regen Braking Algorithm/1(P_elec_W)  "<P_elec_dem_W>"
  Bus Selector/4 -> Unit Delay/1, Unit Delay6/1, Battery Power Limit Calculator/1(<Batt_SOC_frac>), Proposed ReOpt DP Algorithm/1(<Batt_SOC_frac>)  "<Batt_SOC_frac>"
  PropSys_to_EMC/1 -> Bus Selector/1
  From_PCL_BUS/1 -> Bus Selector1/1
  Bus Creator/1 -> EMC_to_PropSys/1
  Power Split - Engine Factor/1 -> Bus Creator/7  "pwrSplitEngFactor"
  Generator Power W/1 -> Bus Creator/8  "P_gen_elec_W"
  Bus Selector/1 -> Rate Transition/1, SPHET Power Mode Selector - Fixed/2(P_veh), SPHET Power Mode Selector - DCARTDP/5(P_veh)  "<P_veh_dem_W>"

== system platooning_custom_blocks/Battery Electric Truck/Battery Electric Post-Processing/Blending Function ==
  runAvgElecEC_Wh_m : Inport
  <Batt_SOC_frac> : Inport  Port=2
  stAvgElecEC_Wh_m : Inport  Port=3
  Constant1 : Constant
  Product1 : Product
  Subtract1 : Sum  Inputs=+-
  Subtract2 : Sum  Inputs=+-
  Subtract3 : Sum  Inputs=+-
  blndElecEC_Wh_m : Outport
  wires:
  runAvgElecEC_Wh_m/1 -> Subtract2/1, Subtract1/1
  Subtract2/1 -> blndElecEC_Wh_m/1  "blndElecEC_Wh_m"
  <Batt_SOC_frac>/1 -> Subtract3/2
  stAvgElecEC_Wh_m/1 -> Subtract1/2
  Subtract3/1 -> Product1/1
  Product1/1 -> Subtract2/2
  Subtract1/1 -> Product1/2
  Constant1/1 -> Subtract3/1

== system platooning_custom_blocks/Battery Electric Truck/Battery Electric Post-Processing/Distance to Empty Calculator ==
  blndEC_Wh_m : Inport
  battSOC_frac : Inport  Port=2
  Battery Energy Max : Constant  Value=msk_batt_Ns * msk_batt_Np * msk_batt_Nmod * msk_cell_Vnom * msk_cell_Q_Ah
  Constant1 : Constant  Value=0.1
  Divide : Product  Inputs=*/
  Product3 : Product
  Subtract1 : Sum  Inputs=+-
  m2km : Gain  Gain=0.001
  estDTE_km : Outport
  wires:
  Divide/1 -> m2km/1
  Product3/1 -> Divide/1
  Subtract1/1 -> Product3/1
  Battery Energy Max/1 -> Product3/2
  battSOC_frac/1 -> Subtract1/1
  Constant1/1 -> Subtract1/2
  blndEC_Wh_m/1 -> Divide/2
  m2km/1 -> estDTE_km/1  "estDTE_km"

== system platooning_custom_blocks/Battery Electric Truck/Battery Electric Powertrain Power Loss Model/A123 ESS Model ==
  Inp_Current : Inport
  Add : Sum  Inputs=++++
  Bus Creator : BusCreator  Inputs=7
  OCV_Battery : Subsystem
  R0 Resistance : Subsystem
  R1_C1 Circuit : Subsystem
  R2_C2 Circuit : Subsystem
  Info : Outport
  Load_Voltage : Outport  Port=2
  SOC : Outport  Port=3
  Current : Outport  Port=4
  wires:
  [SOC] -> Bus Creator/3
  [U_PA] -> Bus Creator/7
  Inp_Current/1 -> OCV_Battery/1(Current)
  [current] -> Bus Creator/2
  Add/1 -> Load_Voltage/1, [V_L]  "V_L"
  [Em] -> Bus Creator/4
  R0 Resistance/1(V_R0) -> [V_R0], Add/3  "V_R0"
  R2_C2 Circuit/1(U_PA) -> Add/1, [U_PA]  "U_PA"
  OCV_Battery/2(Current_pt) -> Current/1, [current], R2_C2 Circuit/2(Current), R1_C1 Circuit/2(Current), R0 Resistance/2(Current)  "Current"
  OCV_Battery/1(SOC_calc) -> SOC/1, [SOC], R2_C2 Circuit/1(SOC), R1_C1 Circuit/1(SOC), R0 Resistance/1(SOC)  "SOC"
  R1_C1 Circuit/1(U_PC) -> Add/2, [U_PC]  "U_PC"
  [U_PC] -> Bus Creator/6
  OCV_Battery/3(BattVolt_calc) -> [Em], Add/4  "Em"
  [V_R0] -> Bus Creator/5
  Bus Creator/1 -> Info/1  "Info"
  [V_L] -> Bus Creator/1

== system platooning_custom_blocks/Battery Electric Truck/Battery Electric Powertrain Power Loss Model/Battery EPO Logic ==
  note: Discharge Current is negative
  Batt_SOC_frac : Inport
  LoadCurrent_A : Inport  Port=2
  10-second average : dspstat3/Moving Average  Method=Sliding window  ForgettingFactorPort=off  SpecifyWindowLength=on  WindowLength=1000  ForgettingFactor=0.9  SimulateUsing=Code generation
  10sec Discharge Limit Table A123 : Lookup_n-D  BreakpointsForDimension1=msk_cellTempbpt  BreakpointsForDimension2=msk_soc_bpt  Table=msk_dchglim10s  InternalRulePriority=Speed  RndMeth=Simplest  InputSameDT=on
  Battery EPO Constraint Logic : Stateflow chart  TreatAsAtomicUnit=on
  CellTemp degC : Constant  Value=25
  Gain1 : Gain  Gain=-1
  Batt_EPO : Outport
  wires:
  Batt_SOC_frac/1 -> 10sec Discharge Limit Table A123/2
  LoadCurrent_A/1 -> 10-second average/1
  Battery EPO Constraint Logic/1(epo_flag) -> Batt_EPO/1  "Batt_EPO"
  10-second average/1 -> Battery EPO Constraint Logic/2(LoadCurr)  "LoadCurrent_10sAvg_A"
  CellTemp degC/1 -> 10sec Discharge Limit Table A123/1
  Gain1/1 -> Battery EPO Constraint Logic/1(DchgCurrLim)
  10sec Discharge Limit Table A123/1 -> Gain1/1

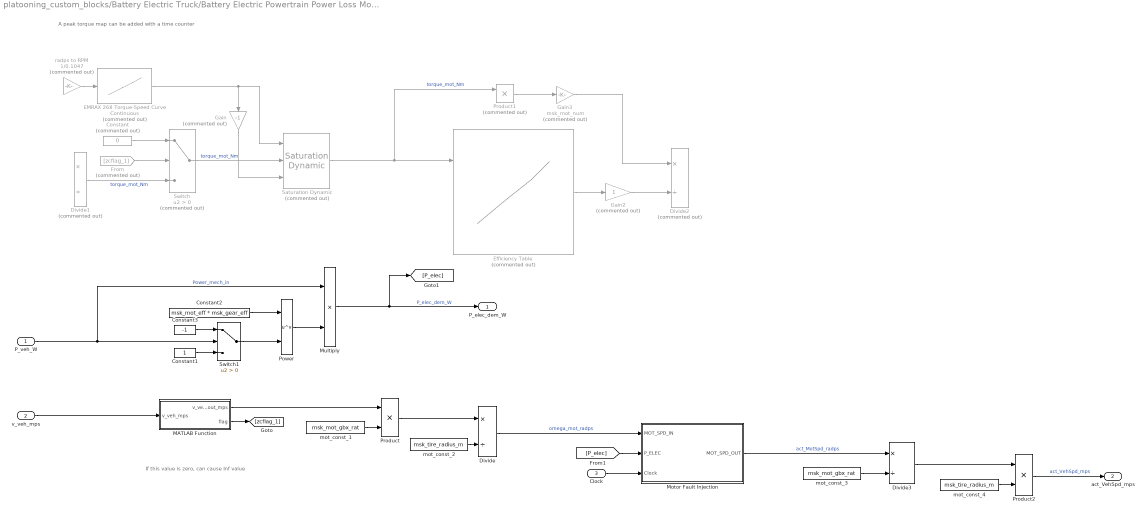
== system platooning_custom_blocks/Battery Electric Truck/Battery Electric Powertrain Power Loss Model/Electric Drivetrain ==
  note: A peak torque map can be added with a time counter
  note: If this value is zero, can cause Inf value
  P_veh_W : Inport
  v_veh_mps : Inport  Port=2
  Clock : Inport  Port=3
  Constant : Constant  Commented=on  Value=0
  Constant1 : Constant
  Constant2 : Constant  Value=msk_mot_eff * msk_gear_eff
  Constant3 : Constant  Value=-1
  Divide : Product  Inputs=*/
  Divide1 : Product  Commented=on  Inputs=*/
  Divide2 : Product  Commented=on  Inputs=*/
  Divide3 : Product  Inputs=*/
  EMRAX 268 Torque-Speed Curve Continuous : Lookup_n-D  Commented=on  NumberOfTableDimensions=1  BreakpointsForDimension1=msk_mot_spd_bpt  Table=msk_mot_cont_trq  InternalRulePriority=Speed  RndMeth=Simplest  InputSameDT=on
  Efficiency Table : Lookup_n-D  Commented=on  BreakpointsForDimension1=motTrqVec  BreakpointsForDimension2=motSpdVec  Table=adj_motEffMap  ExtrapMethod=Clip  UseLastTableValue=on  InternalRulePriority=Speed  RndMeth=Simplest  InputSameDT=on
  From : From  Commented=on  GotoTag=zcflag_1
  Gain : Gain  Commented=on  Gain=-1
  Gain2 : Gain  Commented=on
  Gain3 : Gain  Commented=on  Gain=msk_mot_num
  MATLAB Function : MATLAB Function  TreatAsAtomicUnit=on
  Motor Fault Injection : Subsystem  mask{FaultDec=off, P_derate=30000, t_fault=6000, contMotTrqMax=180}
      mask prompts: FaultDec "Select to enable motor deration fault."; P_derate "Enter the motor deration power [Watts]:"; t_fault "Time for fault insertion [seconds]:"; contMotTrqMax "Maximum Continuous Motor Torque [Nm]:"
      mask DialogControl DescGroupVar Prompt: Motor Fault Injection
      mask DialogControl DescTextVar Prompt: Use the parameter controls to induce a deration fault in the motor subsystem.
  Multiply : Product
  Power : Math  Operator=pow  SaturateOnIntegerOverflow=on
  Product : Product
  Product1 : Product  Commented=on
  Product2 : Product
  Saturation Dynamic : simulink/Discontinuities/Saturation Dynamic  Commented=on  OutMin=[]  OutMax=[]  OutDataTypeStr=Inherit: Same as second input  OutDataType=fixdt(1, 16)  OutScaling=2^-10  DoSatur=off
  Switch : Switch  Commented=on  Criteria=u2 > Threshold
  Switch1 : Switch  Criteria=u2 > Threshold
  mot_const_1 : Constant  Value=msk_mot_gbx_rat
  mot_const_2 : Constant  Value=msk_tire_radius_m
  mot_const_3 : Constant  Value=msk_mot_gbx_rat
  mot_const_4 : Constant  Value=msk_tire_radius_m
  radps to RPM : Gain  Commented=on  Gain=1/0.1047
  P_elec_dem_W : Outport
  act_VehSpd_mps : Outport  Port=2
  wires:
  Saturation Dynamic/1 -> Product1/1, Efficiency Table/1  "torque_mot_Nm"
  From/1 -> Switch/2
  Product/1 -> Divide/1
  radps to RPM/1 -> EMRAX 268 Torque-Speed Curve Continuous/1
  Constant/1 -> Switch/1
  MATLAB Function/1(v_veh_out_mps) -> Product/1
  Gain/1 -> Saturation Dynamic/3
  mot_const_1/1 -> Product/2
  EMRAX 268 Torque-Speed Curve Continuous/1 -> Gain/1, Saturation Dynamic/1
  P_veh_W/1 -> Switch1/2, Multiply/1  "Power_mech_in"
  v_veh_mps/1 -> MATLAB Function/1(v_veh_mps)
  Efficiency Table/1 -> Gain2/1
  Switch/1 -> Saturation Dynamic/2  "torque_mot_Nm"
  mot_const_2/1 -> Divide/2
  MATLAB Function/2(flag) -> [zcflag_1]
  Product1/1 -> Gain3/1
  Multiply/1 -> [P_elec], P_elec_dem_W/1  "P_elec_dem_W"
  Gain2/1 -> Divide2/2
  Gain3/1 -> Divide2/1
  Divide1/1 -> Switch/3  "torque_mot_Nm"
  Motor Fault Injection/1(MOT_SPD_OUT) -> Divide3/1  "act_MotSpd_radps"
  Divide/1 -> Motor Fault Injection/1(MOT_SPD_IN)  "omega_mot_radps"
  [P_elec] -> Motor Fault Injection/2(P_ELEC)
  Clock/1 -> Motor Fault Injection/3(Clock)
  mot_const_3/1 -> Divide3/2
  Divide3/1 -> Product2/1
  mot_const_4/1 -> Product2/2
  Product2/1 -> act_VehSpd_mps/1  "act_VehSpd_mps"
  Constant1/1 -> Switch1/3
  Constant2/1 -> Power/1
  Power/1 -> Multiply/2
  Switch1/1 -> Power/2
  Constant3/1 -> Switch1/1

== system platooning_custom_blocks/Conventional Truck/Conventional Post-Processing/Blending Function 1 ==
  runAvgFuelEC_Wh_m : Inport
  Fuel_Used_L : Inport  Port=2
  stAvgFuelEC_Wh_m : Inport  Port=3
  Constant1 : Constant  Value=msk_fuel_init_liters
  Divide : Product  Inputs=*/
  Product1 : Product
  Subtract1 : Sum  Inputs=-+
  Subtract2 : Sum
  blndElecEC_Wh_m : Outport
  wires:
  Divide/1 -> Product1/1
  runAvgFuelEC_Wh_m/1 -> Subtract1/1, Subtract2/1
  Subtract2/1 -> blndElecEC_Wh_m/1  "blndElecEC_Wh_m"
  stAvgFuelEC_Wh_m/1 -> Subtract1/2
  Fuel_Used_L/1 -> Divide/1
  Product1/1 -> Subtract2/2
  Subtract1/1 -> Product1/2
  Constant1/1 -> Divide/2

== system platooning_custom_blocks/Conventional Truck/Conventional Post-Processing/Blending Function 2 ==
  runAvgFC_L_100km : Inport
  Fuel_Used_L : Inport  Port=2
  stAvgFC_L_100km : Inport  Port=3
  Constant1 : Constant  Value=msk_fuel_init_liters
  Divide : Product  Inputs=*/
  Product1 : Product
  Subtract1 : Sum  Inputs=-+
  Subtract2 : Sum
  blndFC_L_100km : Outport
  wires:
  Subtract1/1 -> Product1/2
  Product1/1 -> Subtract2/2
  stAvgFC_L_100km/1 -> Subtract1/2
  runAvgFC_L_100km/1 -> Subtract1/1, Subtract2/1
  Constant1/1 -> Divide/2
  Fuel_Used_L/1 -> Divide/1
  Divide/1 -> Product1/1
  Subtract2/1 -> blndFC_L_100km/1  "blndFC_L_100km"

== system platooning_custom_blocks/Conventional Truck/Conventional Post-Processing/Distance to Empty Calculator ==
  note: Assuming 10% of the fuel in the tank
      | is not available for consumption.
  blndFC_L_100km : Inport
  <fuelUsed_L> : Inport  Port=2
  Constant : Constant  Value=msk_fuel_init_liters
  Constant2 : Constant  Value=100
  Divide1 : Product  Inputs=*/
  Percent of Fuel in Tank : Gain  Gain=0.9
  Product1 : Product
  Subtract : Sum  Inputs=-+
  estDTE_km : Outport
  wires:
  Percent of Fuel in Tank/1 -> Subtract/2
  blndFC_L_100km/1 -> Divide1/2
  <fuelUsed_L>/1 -> Subtract/1
  Subtract/1 -> Product1/1
  Constant/1 -> Percent of Fuel in Tank/1
  Divide1/1 -> Product1/2  "FC_kmpl"
  Product1/1 -> estDTE_km/1  "estDTE_km"
  Constant2/1 -> Divide1/1

== system platooning_custom_blocks/Conventional Truck/Conventional Post-Processing/Fuel Consumption Calculator ==
  <fuelUsed_L> : Inport
  <DistTrvld_m> : Inport  Port=2
  Constant : Constant  Value=100
  Constant1 : Constant  Value=eps
  Divide1 : Product  Inputs=*/
  Divide2 : Product  Inputs=*/
  Switch : Switch  Criteria=u2 > Threshold
  m2km : Gain  Gain=1/1000
  FC_Lp100km : Outport
  wires:
  Divide2/1 -> FC_Lp100km/1  "FC_Lp100km"
  <DistTrvld_m>/1 -> m2km/1
  Switch/1 -> Divide1/1
  Divide1/1 -> Divide2/2
  m2km/1 -> Switch/1, Switch/2
  <fuelUsed_L>/1 -> Divide1/2
  Constant1/1 -> Switch/3
  Constant/1 -> Divide2/1

== system platooning_custom_blocks/Conventional Truck/Conventional Powertrain Power Loss Model/Engine Torque Saturation ==
  eng_brk_trq : Inport
  eng_spd_rpm : Inport  Port=2
  Engine Peak Motoring Torque LUT : Lookup_n-D  NumberOfTableDimensions=1  BreakpointsForDimension1=eng_spd_bpt  Table=eng_pk_mtr_trq  InternalRulePriority=Speed  RndMeth=Simplest  InputSameDT=on
  "Engine Peak Propulsion Torque LUT " : Lookup_n-D  NumberOfTableDimensions=1  BreakpointsForDimension1=eng_spd_bpt  Table=eng_pk_trq_vec  InternalRulePriority=Speed  RndMeth=Simplest  InputSameDT=on
  Saturation Dynamic : simulink/Discontinuities/Saturation Dynamic  OutMin=[]  OutMax=[]  OutDataTypeStr=Inherit: Same as second input  OutDataType=fixdt(1, 16)  OutScaling=2^-10  DoSatur=off
  eng_brk_trq_out : Outport
  wires:
  eng_brk_trq/1 -> Saturation Dynamic/2
  Saturation Dynamic/1 -> eng_brk_trq_out/1
  eng_spd_rpm/1 -> "Engine Peak Propulsion Torque LUT "/1, Engine Peak Motoring Torque LUT/1
  Engine Peak Motoring Torque LUT/1 -> Saturation Dynamic/3
  "Engine Peak Propulsion Torque LUT "/1 -> Saturation Dynamic/1

== system platooning_custom_blocks/Conventional Truck/Conventional Powertrain Power Loss Model/Fuel Level Calculator ==
  mfuel_gps : Inport
  Constant : Constant  Value=msk_fuel_init_liters
  Discrete-Time Integrator : DiscreteIntegrator  SampleTime=msk_t_step  ICPrevOutput=DiscIntNeverNeededParam  ICPrevScaledInput=DiscIntNeverNeededParam
  Divide1 : Product  Inputs=*/
  Fuel Density : Gain  Gain=(0.001/msk_rho_fuel_kgpL)
  Gain1 : Gain  Gain=100
  Subtract : Sum  Inputs=+-
  fuelLvl_pct : Outport
  fuelUsed_L : Outport  Port=2
  wires:
  Divide1/1 -> Gain1/1
  Subtract/1 -> Divide1/1  "fuelLeft_liters"
  Fuel Density/1 -> fuelUsed_L/1, Subtract/2  "fuelUsed_liters"
  Constant/1 -> Divide1/2, Subtract/1
  Discrete-Time Integrator/1 -> Fuel Density/1  "mfuel_g"
  mfuel_gps/1 -> Discrete-Time Integrator/1
  Gain1/1 -> fuelLvl_pct/1  "fuelLvl_pct"

== system platooning_custom_blocks/Series Parallel Hybrid Electric Truck/Series Parallel Hybrid Electric Post-Processing/Blending Function 1 ==
  runAvgFuelEC_Wh_m : Inport
  Fuel_Used_L : Inport  Port=2
  stAvgFuelEC_Wh_m : Inport  Port=3
  Constant1 : Constant  Value=msk_fuel_init_liters
  Divide : Product  Inputs=*/
  Product1 : Product
  Subtract1 : Sum  Inputs=-+
  Subtract2 : Sum
  blndElecEC_Wh_m : Outport
  wires:
  runAvgFuelEC_Wh_m/1 -> Subtract1/1, Subtract2/1
  stAvgFuelEC_Wh_m/1 -> Subtract1/2
  Divide/1 -> Product1/1
  Fuel_Used_L/1 -> Divide/1
  Constant1/1 -> Divide/2
  Product1/1 -> Subtract2/2
  Subtract1/1 -> Product1/2
  Subtract2/1 -> blndElecEC_Wh_m/1  "blndElecEC_Wh_m"

== system platooning_custom_blocks/Series Parallel Hybrid Electric Truck/Series Parallel Hybrid Electric Post-Processing/Blending Function 2 ==
  runAvgFC_L_100km : Inport
  Fuel_Used_L : Inport  Port=2
  stAvgFC_L_100km : Inport  Port=3
  Constant1 : Constant  Value=msk_fuel_init_liters
  Divide : Product  Inputs=*/
  Product1 : Product
  Subtract1 : Sum  Inputs=-+
  Subtract2 : Sum
  blndFC_L_100km : Outport
  wires:
  Subtract1/1 -> Product1/2
  Product1/1 -> Subtract2/2
  stAvgFC_L_100km/1 -> Subtract1/2
  runAvgFC_L_100km/1 -> Subtract1/1, Subtract2/1
  Constant1/1 -> Divide/2
  Fuel_Used_L/1 -> Divide/1
  Divide/1 -> Product1/1
  Subtract2/1 -> blndFC_L_100km/1  "blndFC_L_100km"
